simulink model "exercise3_model"  (R2015a)
settings: Solver=ode45  StartTime=0.0  StopTime=10.0  RelTol=1e-3
values from neighbouring files (symbols this model uses):
  den = [1 1/R*C 1/L*C]    [exercise1.m]    (also in exercise2.m = [1 1 (1/(R*C) + 2*qp*C)]; exercise3.m = [1 2*Ws_d*zeta_d Ws_d^2])
  kp = ( coef_s - coef_s_lc) /(num_G_s)    [exercise3.m]
  num = [1 0 1/L*C]    [exercise1.m]    (also in exercise2.m = [1/(R*C*L)]; exercise3.m = [gain_d*(Ws_d^2)])
undefined symbols (not defined in the file or in its folder): k1
settings Model: Creator=Daniel Santos  LastModifiedBy=Daniel Santos

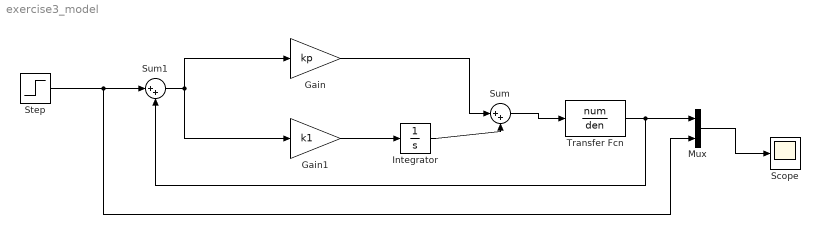
== system exercise3_model ==
  Gain : Gain  Gain=kp
  Gain1 : Gain  Gain=k1
  Integrator : Integrator
  Mux : Mux  Inputs=2
  Scope : Scope
  Step : Step  SampleTime=0
  Sum : Sum  Inputs=|++
  Sum1 : Sum  Inputs=|++
  Transfer Fcn : TransferFcn  Numerator=num  Denominator=den
  wires:
  Step/1 -> Mux/2, Sum1/1
  Sum1/1 -> Gain1/1, Gain/1
  Gain1/1 -> Integrator/1
  Gain/1 -> Sum/1
  Integrator/1 -> Sum/2
  Sum/1 -> Transfer Fcn/1
  Transfer Fcn/1 -> Sum1/2, Mux/1
  Mux/1 -> Scope/1
